simulink model "DFIG_Dynamic_Model1"  (R2013a)
settings: Solver=ode45  StartTime=0.0  StopTime=25  RelTol=1e-3
undefined symbols (not defined in the file): B, C, f, H, Ki, Kp, Lg, Lm, Lr, Ls, P, Pb, sigma, Vb, VDC0, wb, Xm_pu, Xr_pu, Z, Zb
libraries: powerlib_extras x9
settings Model: Creator=Sony  LastModifiedBy=Sony

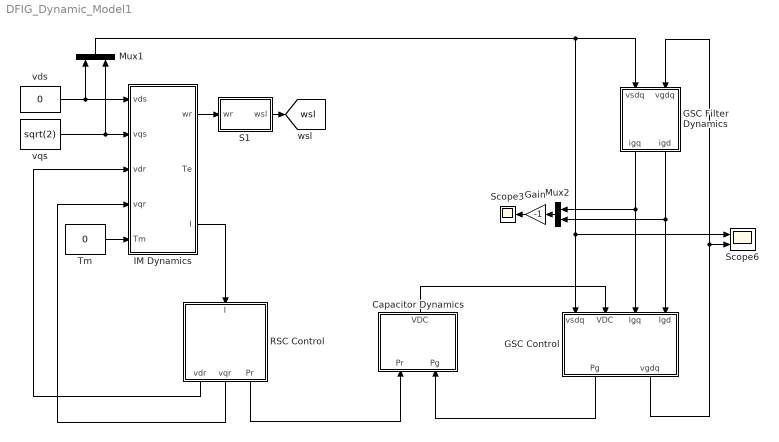
== system DFIG_Dynamic_Model1 ==
  Capacitor Dynamics : Subsystem
  GSC Control : Subsystem
  GSC Filter Dynamics : Subsystem
  Gain : Gain  Gain=-1
  IM Dynamics : Subsystem
  Mux1 : Mux  Inputs=2
  Mux2 : Mux  Inputs=2
  RSC Control : Subsystem
  S1 : Subsystem
  Scope3 : Scope
      settings: YMin=-0.2  YMax=0.2  SaveName=ScopeData10
  Scope6 : Scope  NumInputPorts=2
      settings: YMin=0~0  YMax=1.5~1.5  SaveName=ScopeData16
  Tm : Constant  Value=0
  vds : Constant  Value=0
  vqs : Constant  Value=sqrt(2)
  tag scope: wsl=global
  wires:
  IM Dynamics/3(I) -> RSC Control/1(I)
  Tm/1 -> IM Dynamics/5(Tm)
  vds/1 -> IM Dynamics/1(vds), Mux1/1
  RSC Control/1(vdr) -> IM Dynamics/3(vdr)
  RSC Control/2(vqr) -> IM Dynamics/4(vqr)
  RSC Control/3(Pr) -> Capacitor Dynamics/1(Pr)
  Capacitor Dynamics/1(VDC) -> GSC Control/2(VDC)
  GSC Control/1(Pg) -> Capacitor Dynamics/2(Pg)
  vqs/1 -> IM Dynamics/2(vqs), Mux1/2
  Mux1/1 -> GSC Filter Dynamics/1(vsdq), GSC Control/1(vsdq), Scope6/1
  GSC Control/2(vgdq) -> GSC Filter Dynamics/2(vgdq), Scope6/2
  IM Dynamics/1(wr) -> S1/1(wr)
  S1/1(wsl) -> [wsl]
  Mux2/1 -> Gain/1
  GSC Filter Dynamics/1(igq) -> Mux2/1, GSC Control/3(Igq)
  GSC Filter Dynamics/2(igd) -> Mux2/2, GSC Control/4(Igd)
  Gain/1 -> Scope3/1

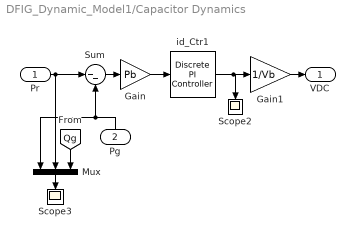
== system DFIG_Dynamic_Model1/Capacitor Dynamics ==
  Pr : Inport
  Pg : Inport  Port=2
  Gain : Gain  Gain=Pb
  Gain1 : Gain  Gain=1/Vb
  Mux : Mux  Inputs=3
  Scope2 : Scope
      settings: YMin=1190  YMax=1230  SaveName=ScopeData5
  Scope3 : Scope
      settings: YMin=-0.5  YMax=0.2  SaveName=ScopeData12
  Sum : Sum  Inputs=|--
  id_Ctr1 : powerlib_extras/Discrete  Control Blocks/Discrete PI Controller  Kp=0  Ki=1/(C*VDC0)  Par_Limits=[10e5 -10e5]  Init=1200  Ts=50e-6
  VDC : Outport
  wires:
  Sum/1 -> Gain/1
  Pr/1 -> Sum/1, Mux/2
  Pg/1 -> Mux/1, Sum/2
  id_Ctr1/1 -> Scope2/1, Gain1/1
  Gain/1 -> id_Ctr1/1
  Gain1/1 -> VDC/1
  [Qg] -> Mux/3
  Mux/1 -> Scope3/1

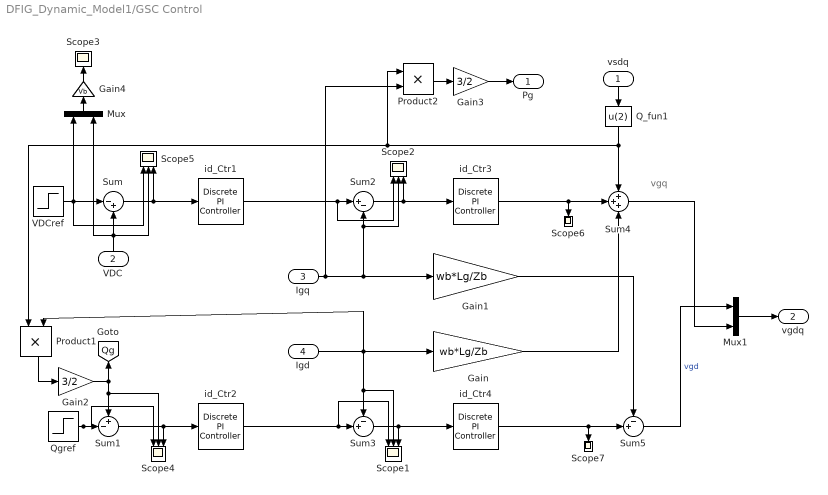
== system DFIG_Dynamic_Model1/GSC Control ==
  note: vgq
  vsdq : Inport
  VDC : Inport  Port=2
  Igq : Inport  Port=3
  Igd : Inport  Port=4
  Gain : Gain  Gain=wb*Lg/Zb
  Gain1 : Gain  Gain=wb*Lg/Zb
  Gain2 : Gain  Gain=3/2
  Gain3 : Gain  Gain=3/2
  Gain4 : Gain  Gain=Vb
  Mux : Mux  Inputs=2
  Mux1 : Mux  Inputs=2
  Product1 : Product
  Product2 : Product
  Q_fun1 : Fcn  Expr=u(2)
  Qgref : Step  After=0  SampleTime=0
  Scope{1..2,4..5} (4 alike) : Scope  NumInputPorts=3
      Scope1 settings: YMin=-15~-15~-0.1  YMax=5~5~0.1  SaveName=ScopeData6
      Scope2 settings: YMin=-0.5~-0.5~-0.1  YMax=0.1~0.5~0.1  SaveName=ScopeData2
      Scope4 settings: YMin=-1~-0.5~-0.5  YMax=1~0.5~0.5  SaveName=ScopeData9
      Scope5 settings: YMin=3~3.01~-0.055  YMax=3.07~3.065~0.055  SaveName=ScopeData11
  Scope3 : Scope
      settings: YMin=1195  YMax=1225  SaveName=ScopeData22
  Scope6 : Scope
      settings: YMin=-1  YMax=1  SaveName=ScopeData24
  Scope7 : Scope
      settings: YMin=-1  YMax=1  SaveName=ScopeData25
  Sum : Sum  Inputs=|-+
  Sum1 : Sum  Inputs=+-|
  Sum2 : Sum  Inputs=|+-
  Sum3 : Sum  Inputs=-+|
  Sum4 : Sum  Inputs=+++
  Sum5 : Sum  Inputs=-+|
  VDCref : Step  Time=20  Before=1200/Vb  After=1220/Vb  SampleTime=0
  id_Ctr1 : powerlib_extras/Discrete  Control Blocks/Discrete PI Controller  Kp=Kp  Ki=Ki  Par_Limits=[10e5 -10e5]  Init=0  Ts=50e-6
  id_Ctr2 : powerlib_extras/Discrete  Control Blocks/Discrete PI Controller  Kp=Kp  Ki=Ki  Par_Limits=[10e5 -10e5]  Init=-0.0301  Ts=50e-6
  id_Ctr3 : powerlib_extras/Discrete  Control Blocks/Discrete PI Controller  Kp=Kp  Ki=Ki  Par_Limits=[10e5 -10e5]  Init=0  Ts=50e-6
  id_Ctr4 : powerlib_extras/Discrete  Control Blocks/Discrete PI Controller  Kp=Kp  Ki=Ki  Par_Limits=[10e5 -10e5]  Init=0  Ts=50e-6
  Pg : Outport
  vgdq : Outport  Port=2
  tag scope: Qg=global
  wires:
  VDCref/1 -> Scope5/1, Sum/1, Mux/1
  VDC/1 -> Mux/2, Scope5/2, Sum/2
  Qgref/1 -> Scope4/1, Sum1/2
  Gain2/1 -> Scope4/2, Sum1/1, [Qg]
  Q_fun1/1 -> Product1/1, Product2/1, Sum4/1
  Sum3/1 -> id_Ctr4/1, Scope1/3
  Sum2/1 -> id_Ctr3/1, Scope2/3
  Sum1/1 -> Scope4/3, id_Ctr2/1
  id_Ctr1/1 -> Sum2/1, Scope2/1
  id_Ctr4/1 -> Scope7/1, Sum5/2
  Igd/1 -> Product1/2, Sum3/1, Scope1/2, Gain/1
  id_Ctr2/1 -> Scope1/1, Sum3/2
  id_Ctr3/1 -> Scope6/1, Sum4/2
  Product1/1 -> Gain2/1
  Product2/1 -> Gain3/1
  Gain3/1 -> Pg/1
  Sum/1 -> id_Ctr1/1, Scope5/3
  Gain1/1 -> Sum5/1
  Gain/1 -> Sum4/3
  Mux/1 -> Gain4/1
  vsdq/1 -> Q_fun1/1
  Mux1/1 -> vgdq/1
  Sum5/1 -> Mux1/1  "vgd"
  Sum4/1 -> Mux1/2
  Gain4/1 -> Scope3/1
  Igq/1 -> Gain1/1, Scope2/2, Sum2/2, Product2/2

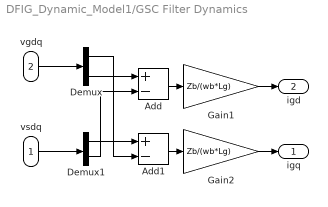
== system DFIG_Dynamic_Model1/GSC Filter Dynamics ==
  vsdq : Inport
  vgdq : Inport  Port=2
  Add : Sum  Inputs=+-
  Add1 : Sum  Inputs=+-
  Demux : Demux  Outputs=2
  Demux1 : Demux  Outputs=2
  Gain1 : Gain  Gain=Zb/(wb*Lg)
  Gain2 : Gain  Gain=Zb/(wb*Lg)
  igq : Outport
  igd : Outport  Port=2
  wires:
  vsdq/1 -> Demux1/1
  Add/1 -> Gain1/1
  vgdq/1 -> Demux/1
  Gain1/1 -> igd/1
  Gain2/1 -> igq/1
  Add1/1 -> Gain2/1
  Demux/2 -> Add/1
  Demux1/2 -> Add/2
  Demux1/1 -> Add1/1
  Demux/1 -> Add1/2

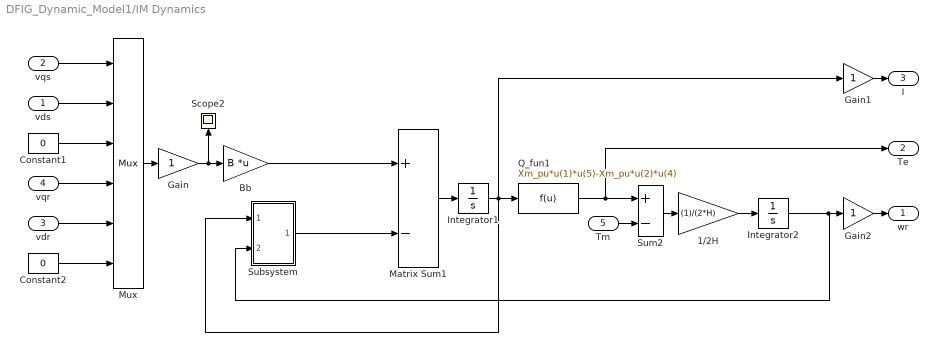
== system DFIG_Dynamic_Model1/IM Dynamics ==
  vds : Inport
  vqs : Inport  Port=2
  vdr : Inport  Port=3
  vqr : Inport  Port=4
  Tm : Inport  Port=5
  1/2H : Gain  Gain=(1)/(2*H)
  Bb : Gain  Gain=B  Multiplication=Matrix(K*u)
  Constant1 : Constant  Value=0
  Constant2 : Constant  Value=0
  Gain : Gain
  Gain1 : Gain
  Gain2 : Gain
  Integrator1 : Integrator  InitialCondition=[-0.57; 0; 0; 0.57; 0.358; 0]
  Integrator2 : Integrator  InitialCondition=0.95  LimitOutput=on  UpperSaturationLimit=0.95000000001  LowerSaturationLimit=0.94999999999
  Matrix Sum1 : Sum  Inputs=+-
  Mux : Mux  Inputs=6
  Q_fun1 : Fcn  Expr=Xm_pu*u(1)*u(5)-Xm_pu*u(2)*u(4)
  Scope2 : Scope
      settings: YMin=950000  YMax=1.05e+06  SaveName=ScopeData8
  Subsystem : Subsystem
  Sum2 : Sum  Inputs=+-  SaturateOnIntegerOverflow=on  InputSameDT=on  OutDataTypeStr=Inherit: Same as first input
  wr : Outport
  Te : Outport  Port=2
  I : Outport  Port=3
  wires:
  Sum2/1 -> 1/2H/1
  vqs/1 -> Mux/1
  Matrix Sum1/1 -> Integrator1/1
  Constant1/1 -> Mux/3
  Tm/1 -> Sum2/2
  Q_fun1/1 -> Te/1, Sum2/1
  vds/1 -> Mux/2
  vdr/1 -> Mux/5
  Gain/1 -> Scope2/1, Bb/1
  vqr/1 -> Mux/4
  1/2H/1 -> Integrator2/1
  Integrator1/1 -> Gain1/1, Subsystem/1(In1), Q_fun1/1
  Bb/1 -> Matrix Sum1/1
  Integrator2/1 -> Subsystem/2(In2), Gain2/1
  Subsystem/1(Out1) -> Matrix Sum1/2
  Constant2/1 -> Mux/6
  Mux/1 -> Gain/1
  Gain1/1 -> I/1
  Gain2/1 -> wr/1

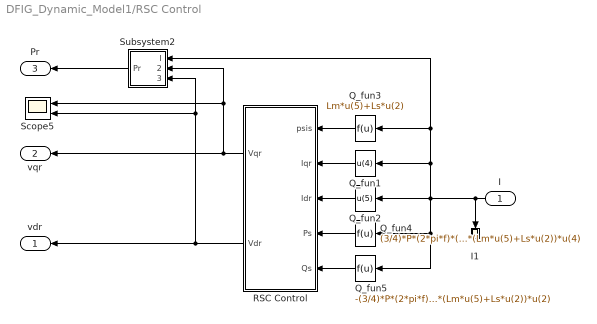
== system DFIG_Dynamic_Model1/RSC Control ==
  I : Inport
  I1 : Scope
      settings: YMin=-1  YMax=1
  Q_fun1 : Fcn  Expr=u(4)
  Q_fun2 : Fcn  Expr=u(5)
  Q_fun3 : Fcn  Expr=Lm*u(5)+Ls*u(2)
  Q_fun4 : Fcn  Expr=(3/4)*P*(2*pi*f)*(Lm/Ls)*(Lm*u(5)+Ls*u(2))*u(4)
  Q_fun5 : Fcn  Expr=-(3/4)*P*(2*pi*f)*(Lm*u(5)+Ls*u(2))*u(2)
  RSC Control : Subsystem
  Scope5 : Scope  NumInputPorts=2
      settings: YMin=-1~-1  YMax=1~1  SaveName=ScopeData15
  Subsystem2 : Subsystem
  vdr : Outport
  vqr : Outport  Port=2
  Pr : Outport  Port=3
  wires:
  Subsystem2/1(Pr) -> Pr/1
  RSC Control/2(Vdr) -> vdr/1, Subsystem2/3(vdr), Scope5/2
  Q_fun3/1 -> RSC Control/1(psis)
  Q_fun4/1 -> RSC Control/4(Ps)
  RSC Control/1(Vqr) -> vqr/1, Subsystem2/2(vqr), Scope5/1
  Q_fun2/1 -> RSC Control/3(Idr)
  Q_fun1/1 -> RSC Control/2(Iqr)
  Q_fun5/1 -> RSC Control/5(Qs)
  I/1 -> Subsystem2/1(I), Q_fun3/1, Q_fun1/1, Q_fun5/1, Q_fun4/1, Q_fun2/1, I1/1

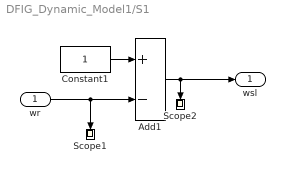
== system DFIG_Dynamic_Model1/S1 ==
  wr : Inport
  Add1 : Sum  Inputs=+-
  Constant1 : Constant
  Scope1 : Scope
      settings: YMin=0.9025  YMax=0.9975  SaveName=ScopeData13
  Scope2 : Scope
      settings: YMin=0.0475  YMax=0.0525  SaveName=ScopeData18
  wsl : Outport
  wires:
  Constant1/1 -> Add1/1
  wr/1 -> Scope1/1, Add1/2
  Add1/1 -> wsl/1, Scope2/1

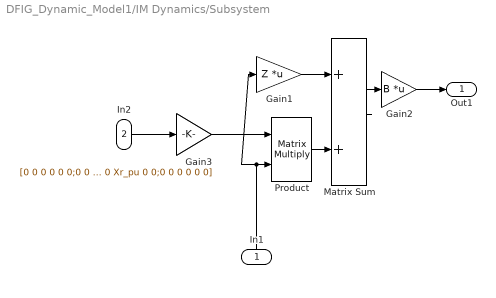
== system DFIG_Dynamic_Model1/IM Dynamics/Subsystem ==
  In1 : Inport
  In2 : Inport  Port=2
  Gain1 : Gain  Gain=Z  Multiplication=Matrix(K*u)
  Gain2 : Gain  Gain=B  Multiplication=Matrix(K*u)
  Gain3 : Gain  Gain=[0 0 0 0 0 0;0 0 0 0 0 0;0 0 0 0 0 0;0 -Xm_pu 0 0 -Xr_pu 0;Xm_pu 0 0 Xr_pu 0 0;0 0 0 0 0 0]
  Matrix Sum : Sum
  Product : Product  Multiplication=Matrix(*)
  Out1 : Outport
  wires:
  Gain2/1 -> Out1/1
  Product/1 -> Matrix Sum/2
  Matrix Sum/1 -> Gain2/1
  Gain3/1 -> Product/1
  Gain1/1 -> Matrix Sum/1
  In1/1 -> Gain1/1, Product/2
  In2/1 -> Gain3/1

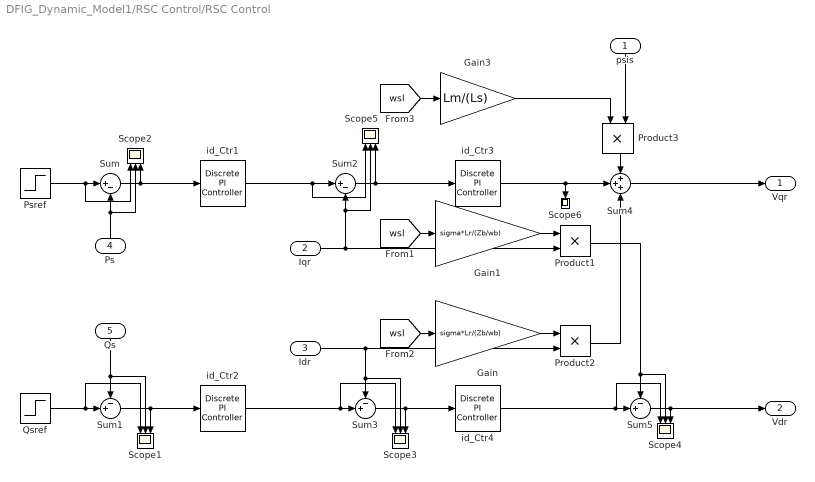
== system DFIG_Dynamic_Model1/RSC Control/RSC Control ==
  psis : Inport
  Iqr : Inport  Port=2
  Idr : Inport  Port=3
  Ps : Inport  Port=4
  Qs : Inport  Port=5
  Gain : Gain  Gain=sigma*Lr/(Zb/wb)
  Gain1 : Gain  Gain=sigma*Lr/(Zb/wb)
  Gain3 : Gain  Gain=Lm/(Ls)
  Product1 : Product
  Product2 : Product
  Product3 : Product
  Psref : Step  Before=0.95*0.95*0.95  After=0.95*0.95*0.95  SampleTime=0
  Qsref : Step  After=0  SampleTime=0
  Scope{1..5} (5 alike) : Scope  NumInputPorts=3
      Scope1 settings: YMin=-1~-1~-0.1  YMax=1~1~0.1  SaveName=ScopeData4
      Scope2 settings: YMin=0.814506~0.814506~-0.2  YMax=0.900244~0.900244~0.2  SaveName=ScopeData3
      Scope3 settings: YMin=0.241271~0.241271~-0.1  YMax=0.266668~0.266668~0.1  SaveName=ScopeData7
      Scope4 settings: YMin=0.00132459~0.00735382~-0.00666389  YMax=0.00146401~0.0081279~-0.00602923  SaveName=ScopeData17
      Scope5 settings: YMin=0.578025~0.578034~-1.25e-05  YMax=0.578047~0.578038~1.25e-05  SaveName=ScopeData20
  Scope6 : Scope
      settings: YMin=-1  YMax=1
  Sum : Sum  Inputs=|+-
  Sum1 : Sum  Inputs=-+|
  Sum2 : Sum  Inputs=|+-
  Sum3 : Sum  Inputs=-+|
  Sum4 : Sum  Inputs=+++
  Sum5 : Sum  Inputs=-+|
  id_Ctr1 : powerlib_extras/Discrete  Control Blocks/Discrete PI Controller  Kp=Kp  Ki=Ki  Par_Limits=[10e5 -10e5]  Init=0.578  Ts=50e-6
  id_Ctr2 : powerlib_extras/Discrete  Control Blocks/Discrete PI Controller  Kp=Kp  Ki=Ki  Par_Limits=[10e5 -10e5]  Init=0.3585  Ts=50e-6
  id_Ctr3 : powerlib_extras/Discrete  Control Blocks/Discrete PI Controller  Kp=Kp  Ki=Ki  Par_Limits=[10e5 -10e5]  Init=0.0723  Ts=50e-6
  id_Ctr4 : powerlib_extras/Discrete  Control Blocks/Discrete PI Controller  Kp=Kp  Ki=Ki  Par_Limits=[10e5 -10e5]  Init=0.00198  Ts=50e-6
  Vqr : Outport
  Vdr : Outport  Port=2
  wires:
  Psref/1 -> Scope2/1, Sum/1
  Ps/1 -> Scope2/2, Sum/2
  Qsref/1 -> Scope1/1, Sum1/2
  Qs/1 -> Scope1/2, Sum1/1
  Sum/1 -> id_Ctr1/1, Scope2/3
  Product3/1 -> Sum4/1
  Sum3/1 -> Scope3/3, id_Ctr4/1
  Gain1/1 -> Product1/1
  Sum2/1 -> id_Ctr3/1, Scope5/3
  Sum1/1 -> Scope1/3, id_Ctr2/1
  id_Ctr4/1 -> Scope4/1, Sum5/2
  Iqr/1 -> Scope5/2, Sum2/2, Product1/2
  Idr/1 -> Scope3/2, Sum3/1, Product2/2
  id_Ctr2/1 -> Scope3/1, Sum3/2
  id_Ctr3/1 -> Scope6/1, Sum4/2
  Gain/1 -> Product2/1
  Sum4/1 -> Vqr/1
  Sum5/1 -> Scope4/3, Vdr/1
  [wsl] -> Gain1/1
  [wsl] -> Gain/1
  Product1/1 -> Scope4/2, Sum5/1
  Product2/1 -> Sum4/3
  Gain3/1 -> Product3/1
  psis/1 -> Product3/2
  [wsl] -> Gain3/1
  id_Ctr1/1 -> Scope5/1, Sum2/1

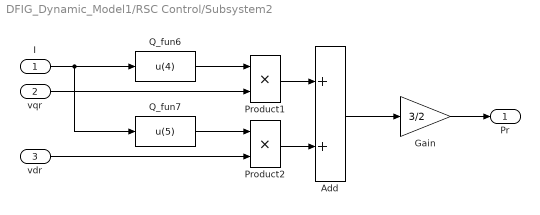
== system DFIG_Dynamic_Model1/RSC Control/Subsystem2 ==
  I : Inport
  vqr : Inport  Port=2
  vdr : Inport  Port=3
  Add : Sum
  Gain : Gain  Gain=3/2
  Product1 : Product
  Product2 : Product
  Q_fun6 : Fcn  Expr=u(4)
  Q_fun7 : Fcn  Expr=u(5)
  Pr : Outport
  wires:
  Product2/1 -> Add/2
  Gain/1 -> Pr/1
  Q_fun6/1 -> Product1/1
  I/1 -> Q_fun7/1, Q_fun6/1
  Product1/1 -> Add/1
  Q_fun7/1 -> Product2/1
  vdr/1 -> Product2/2
  vqr/1 -> Product1/2
  Add/1 -> Gain/1
